simulink model "SS_IEEE_9_bus_revised_dynamicPhasor1"  (R2023b)
settings: Solver=VariableStepAuto  StartTime=0.0  StopTime=10.0  RelTol=1e-3
settings Model: Creator=dongyuli  LastModifiedBy=dongyuli

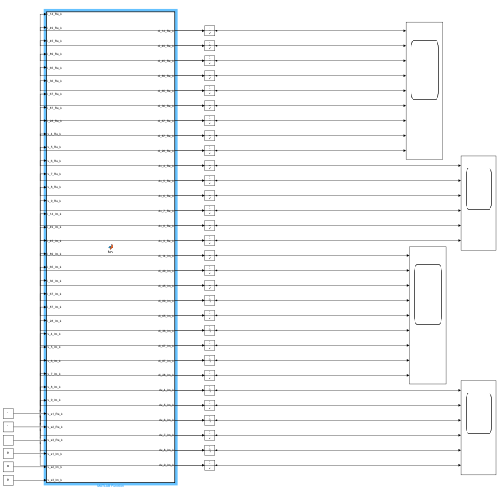
[thumbnail: Simulink's stored preview of the top-level diagram]
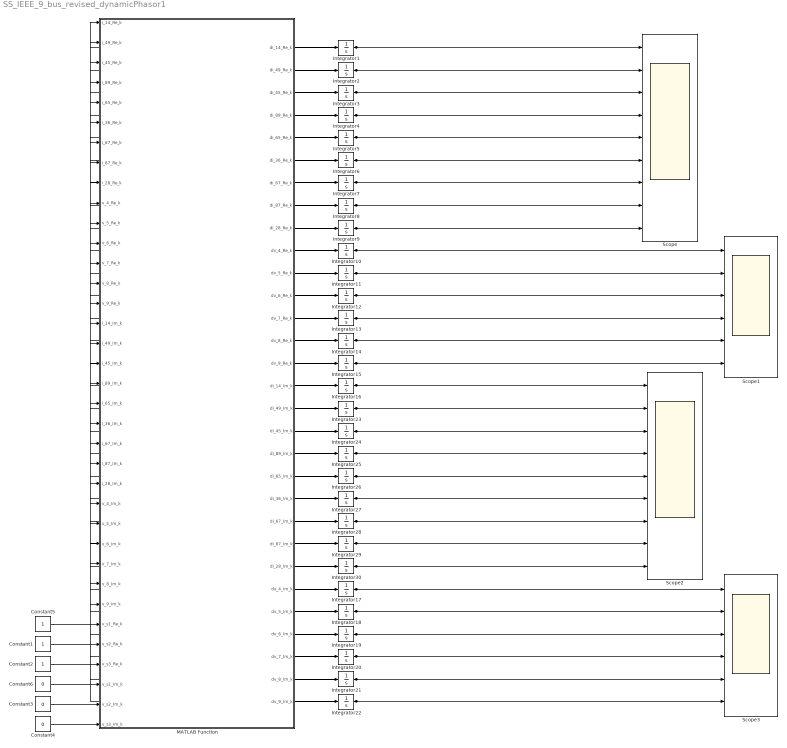
== system SS_IEEE_9_bus_revised_dynamicPhasor1 ==
  Constant1 : Constant
  Constant2 : Constant
  Constant3 : Constant  Value=0
  Constant4 : Constant  Value=0
  Constant5 : Constant
  Constant6 : Constant  Value=0
  Integrator{1..30} (30 alike) : Integrator
  MATLAB Function : MATLAB Function  TreatAsAtomicUnit=on
  Scope : Scope  NumInputPorts=9
  Scope1 : Scope  NumInputPorts=6
  Scope2 : Scope  NumInputPorts=9
  Scope3 : Scope  NumInputPorts=6
  wires:
  MATLAB Function/1(di_14_Re_k) -> Integrator1/1
  MATLAB Function/2(di_49_Re_k) -> Integrator2/1
  MATLAB Function/3(di_45_Re_k) -> Integrator3/1
  MATLAB Function/4(di_89_Re_k) -> Integrator4/1
  MATLAB Function/5(di_65_Re_k) -> Integrator5/1
  MATLAB Function/6(di_36_Re_k) -> Integrator6/1
  MATLAB Function/7(di_67_Re_k) -> Integrator7/1
  MATLAB Function/8(di_87_Re_k) -> Integrator8/1
  MATLAB Function/9(di_28_Re_k) -> Integrator9/1
  MATLAB Function/10(dv_4_Re_k) -> Integrator10/1
  MATLAB Function/11(dv_5_Re_k) -> Integrator11/1
  MATLAB Function/12(dv_6_Re_k) -> Integrator12/1
  MATLAB Function/13(dv_7_Re_k) -> Integrator13/1
  MATLAB Function/14(dv_8_Re_k) -> Integrator14/1
  MATLAB Function/15(dv_9_Re_k) -> Integrator15/1
  MATLAB Function/16(di_14_Im_k) -> Integrator16/1
  MATLAB Function/17(di_49_Im_k) -> Integrator23/1
  MATLAB Function/18(di_45_Im_k) -> Integrator24/1
  MATLAB Function/19(di_89_Im_k) -> Integrator25/1
  MATLAB Function/20(di_65_Im_k) -> Integrator26/1
  MATLAB Function/21(di_36_Im_k) -> Integrator27/1
  MATLAB Function/22(di_67_Im_k) -> Integrator28/1
  MATLAB Function/23(di_87_Im_k) -> Integrator29/1
  MATLAB Function/24(di_28_Im_k) -> Integrator30/1
  MATLAB Function/25(dv_4_Im_k) -> Integrator17/1
  MATLAB Function/26(dv_5_Im_k) -> Integrator18/1
  MATLAB Function/27(dv_6_Im_k) -> Integrator19/1
  MATLAB Function/28(dv_7_Im_k) -> Integrator20/1
  MATLAB Function/29(dv_8_Im_k) -> Integrator21/1
  MATLAB Function/30(dv_9_Im_k) -> Integrator22/1
  Integrator1/1 -> Scope/1, MATLAB Function/1(i_14_Re_k)
  Integrator2/1 -> Scope/2, MATLAB Function/2(i_49_Re_k)
  Integrator3/1 -> Scope/3, MATLAB Function/3(i_45_Re_k)
  Constant5/1 -> MATLAB Function/31(v_s1_Re_k)
  Constant1/1 -> MATLAB Function/32(v_s2_Re_k)
  Constant2/1 -> MATLAB Function/33(v_s3_Re_k)
  Integrator4/1 -> Scope/4, MATLAB Function/4(i_89_Re_k)
  Integrator5/1 -> Scope/5, MATLAB Function/5(i_65_Re_k)
  Integrator6/1 -> Scope/6, MATLAB Function/6(i_36_Re_k)
  Integrator7/1 -> Scope/7, MATLAB Function/7(i_67_Re_k)
  Integrator8/1 -> Scope/8, MATLAB Function/8(i_87_Re_k)
  Integrator9/1 -> Scope/9, MATLAB Function/9(i_28_Re_k)
  Integrator10/1 -> Scope1/1, MATLAB Function/10(v_4_Re_k)
  Integrator11/1 -> Scope1/2, MATLAB Function/11(v_5_Re_k)
  Integrator12/1 -> Scope1/3, MATLAB Function/12(v_6_Re_k)
  Integrator13/1 -> Scope1/4, MATLAB Function/13(v_7_Re_k)
  Integrator14/1 -> Scope1/5, MATLAB Function/14(v_8_Re_k)
  Integrator15/1 -> Scope1/6, MATLAB Function/15(v_9_Re_k)
  Integrator16/1 -> Scope2/1, MATLAB Function/16(i_14_Im_k)
  Integrator23/1 -> Scope2/2, MATLAB Function/17(i_49_Im_k)
  Integrator24/1 -> Scope2/3, MATLAB Function/18(i_45_Im_k)
  Integrator25/1 -> Scope2/4, MATLAB Function/19(i_89_Im_k)
  Integrator26/1 -> Scope2/5, MATLAB Function/20(i_65_Im_k)
  Integrator27/1 -> Scope2/6, MATLAB Function/21(i_36_Im_k)
  Integrator28/1 -> Scope2/7, MATLAB Function/22(i_67_Im_k)
  Integrator29/1 -> Scope2/8, MATLAB Function/23(i_87_Im_k)
  Integrator30/1 -> Scope2/9, MATLAB Function/24(i_28_Im_k)
  Integrator17/1 -> Scope3/1, MATLAB Function/25(v_4_Im_k)
  Integrator18/1 -> Scope3/2, MATLAB Function/26(v_5_Im_k)
  Integrator19/1 -> Scope3/3, MATLAB Function/27(v_6_Im_k)
  Integrator20/1 -> Scope3/4, MATLAB Function/28(v_7_Im_k)
  Integrator21/1 -> Scope3/5, MATLAB Function/29(v_8_Im_k)
  Integrator22/1 -> Scope3/6, MATLAB Function/30(v_9_Im_k)
  Constant6/1 -> MATLAB Function/34(v_s1_Im_k)
  Constant3/1 -> MATLAB Function/35(v_s2_Im_k)
  Constant4/1 -> MATLAB Function/36(v_s3_Im_k)

== matlab function SS_IEEE_9_bus_revised_dynamicPhasor1/MATLAB Function ==
  data: i_14_Re_k input; di_14_Re_k output; di_49_Re_k output; di_45_Re_k output; di_89_Re_k output; di_65_Re_k output; di_36_Re_k output; di_67_Re_k output; di_87_Re_k output; di_28_Re_k output; dv_4_Re_k output; dv_5_Re_k output; dv_6_Re_k output; dv_7_Re_k output; dv_8_Re_k output; dv_9_Re_k output; i_49_Re_k input; i_45_Re_k input; i_89_Re_k input; i_65_Re_k input; i_36_Re_k input; i_67_Re_k input; i_87_Re_k input; i_28_Re_k input; v_4_Re_k input; v_5_Re_k input; v_6_Re_k input; v_7_Re_k input; v_8_Re_k input; v_9_Re_k input; i_14_Im_k input; i_49_Im_k input; i_45_Im_k input; i_89_Im_k input; i_65_Im_k input; i_36_Im_k input; i_67_Im_k input; i_87_Im_k input; i_28_Im_k input; v_4_Im_k input; v_5_Im_k input; v_6_Im_k input; v_7_Im_k input; v_8_Im_k input; v_9_Im_k input; v_s1_Re_k input; v_s2_Re_k input; v_s3_Re_k input; di_14_Im_k output; di_49_Im_k output; di_45_Im_k output; di_89_Im_k output; di_65_Im_k output; di_36_Im_k output; di_67_Im_k output; di_87_Im_k output; di_28_Im_k output; dv_4_Im_k output; dv_5_Im_k output; dv_6_Im_k output; dv_7_Im_k output; dv_8_Im_k output; dv_9_Im_k output; v_s1_Im_k input; v_s2_Im_k input; v_s3_Im_k input
function [di_14_Re_k, di_49_Re_k, di_45_Re_k, di_89_Re_k, di_65_Re_k, di_36_Re_k, di_67_Re_k, di_87_Re_k, di_28_Re_k, dv_4_Re_k, dv_5_Re_k, dv_6_Re_k, dv_7_Re_k, dv_8_Re_k, dv_9_Re_k, di_14_Im_k, di_49_Im_k, di_45_Im_k, di_89_Im_k, di_65_Im_k, di_36_Im_k, di_67_Im_k, di_87_Im_k, di_28_Im_k, dv_4_Im_k, dv_5_Im_k, dv_6_Im_k, dv_7_Im_k, dv_8_Im_k, dv_9_Im_k] = fcn(i_14_Re_k, i_49_Re_k, i_45_Re_k, i_89_Re_k, i_65_Re_k, i_36_Re_k, i_67_Re_k, i_87_Re_k, i_28_Re_k, v_4_Re_k, v_5_Re_k, v_6_Re_k, v_7_Re_k, v_8_Re_k, v_9_Re_k, i_14_Im_k, i_49_Im_k, i_45_Im_k, i_89_Im_k, i_65_Im_k, i_36_Im_k, i_67_Im_k, i_87_Im_k, i_28_Im_k, v_4_Im_k, v_5_Im_k, v_6_Im_k, v_7_Im_k, v_8_Im_k, v_9_Im_k, v_s1_Re_k, v_s2_Re_k, v_s3_Re_k, v_s1_Im_k, v_s2_Im_k, v_s3_Im_k)

f = 50;
w = 2*pi*f;

V_base = 345;
MVA_base = 100;
Z_base = (sqrt(3)*V_base^2)/MVA_base;

R_14 = 0.01*Z_base;
R_28 = 0.01*Z_base;
R_36 = 0.01*Z_base;

R_49 = 0.01*Z_base;
R_45 = 0.017*Z_base;
R_89 = 0.032*Z_base;
R_65 = 0.039*Z_base;
R_67 = 0.0119*Z_base;
R_87 = 0.0085*Z_base;

L_14 = 0.0576*Z_base/w;
L_49 = 0.085*Z_base/w;
L_45 = 0.092*Z_base/w;
L_89 = 0.161*Z_base/w;
L_65 = 0.170*Z_base/w;
L_36 = 0.0586*Z_base/w;
L_67 = 0.1008*Z_base/w;
L_87 = 0.072*Z_base/w;
L_28 = 0.0625*Z_base/w;

L_1 = 0.0608*Z_base/w;
L_2 = 0.1198*Z_base/w;
L_3 = 0.1813*Z_base/w;

C_4 = (0.079 + 0.088)*Z_base/w;
C_5 = (0.079 + 0.179)*Z_base/w;
C_6 = (0.179 + 0.1045)*Z_base/w;
C_7 = (0.1045 + 0.0745)*Z_base/w;
C_8 = (0.0745 + 0.153)*Z_base/w;
C_9 = (0.088 + 0.153)*Z_base/w;

X = [i_14_Re_k, i_49_Re_k, i_45_Re_k, i_89_Re_k, i_65_Re_k, i_36_Re_k, i_67_Re_k, i_87_Re_k, i_28_Re_k, v_4_Re_k, v_5_Re_k, v_6_Re_k, v_7_Re_k, v_8_Re_k, v_9_Re_k, i_14_Im_k, i_49_Im_k, i_45_Im_k, i_89_Im_k, i_65_Im_k, i_36_Im_k, i_67_Im_k, i_87_Im_k, i_28_Im_k, v_4_Im_k, v_5_Im_k, v_6_Im_k, v_7_Im_k, v_8_Im_k, v_9_Im_k]';

U = [v_s1_Re_k, v_s2_Re_k, v_s3_Re_k, v_s1_Im_k, v_s2_Im_k, v_s3_Im_k]';

%A =[-R_14/L_14 0 0 0 0 0 0 0 0 1/L_14 0 0 -1/L_14 0 0 0 0 0;
%    0 -R_49/L_49 0 0 0 0 0 0 0 0 0 0 1/L_49 0 0 0 0 -1/L_49;
%    0 0 -R_45/L_45 0 0 0 0 0 0 0 0 0 1/L_45 -1/L_45 0 0 0 0;
%    0 0 0 -R_89/L_89 0 0 0 0 0 0 0 0 0 0 0 0 1/L_89 -1/L_89;
%    0 0 0 0 -R_65/L_65 0 0 0 0 0 0 0 0 -1/L_65 1/L_65 0 0 0;
%    0 0 0 0 0 -R_36/L_36 0 0 0 0 0 1/L_36 0 0 -1/L_36 0 0 0;
%    0 0 0 0 0 0 -R_67/L_67 0 0 0 0 0 0 0 1/L_67 -1/L_67 0 0;
%    0 0 0 0 0 0 0 -R_87/L_87 0 0 0 0 0 0 0 -1/L_87 1/L_87 0;
%    0 0 0 0 0 0 0 0 -R_28/L_28 0 1/L_28 0 0 0 0 0 -1/L_28 0;
%    -1/C_1 0 0 0 0 0 0 0 0 0 0 0 0 0 0 0 0 0;
%    0 0 0 0 0 0 0 0 -1/C_2 0 0 0 0 0 0 0 0 0;
%    0 0 0 0 0 -1/C_3 0 0 0 0 0 0 0 0 0 0 0 0;
%    1/C_4 -1/C_4 -1/C_4 0 0 0 0 0 0 0 0 0 0 0 0 0 0 0;
%    0 0 1/C_5 0 1/C_5 0 0 0 0 0 0 0 0 0 0 0 0 0;
%    0 0 0 0 -1/C_6 1/C_6 -1/C_6 0 0 0 0 0 0 0 0 0 0 0;
%    0 0 0 0 0 0 1/C_7 1/C_7 0 0 0 0 0 0 0 0 0 0;
%    0 0 0 -1/C_8 0 0 0 -1/C_8 1/C_8 0 0 0 0 0 0 0 0 0;
%    0 1/C_9 0 1/C_9 0 0 0 0 0 0 0 0 0 0 0 0 0 0];

A = [-R_14/(L_14+L_1) 0 0 0 0 0 0 0 0 -1/(L_14+L_1) 0 0 0 0 0;
    0 -R_49/L_49 0 0 0 0 0 0 0 1/L_49 0 0 0 0 -1/L_49;
    0 0 -R_45/L_45 0 0 0 0 0 0 1/L_45 -1/L_45 0 0 0 0;
    0 0 0 -R_89/L_89 0 0 0 0 0 0 0 0 0 1/L_89 -1/L_89;
    0 0 0 0 -R_65/L_65 0 0 0 0 0 -1/L_65 1/L_65 0 0 0;
    0 0 0 0 0 -R_36/(L_36+L_3) 0 0 0 0 0 -1/(L_36+L_3) 0 0 0;
    0 0 0 0 0 0 -R_67/L_67 0 0 0 0 1/L_67 -1/L_67 0 0;
    0 0 0 0 0 0 0 -R_87/L_87 0 0 0 0 0 -1/L_87 1/L_87;
    0 0 0 0 0 0 0 0 -R_28/(L_28+L_2) 0 0 0 0 -1/(L_28+L_2) 0;
    1/C_4 -1/C_4 -1/C_4 0 0 0 0 0 0 0 0 0 0 0 0;
    0 0 1/C_5 0 1/C_5 0 0 0 0 0 0 0 0 0 0;
    0 0 0 0 -1/C_6 1/C_6 -1/C_6 0 0 0 0 0 0 0 0;
    0 0 0 0 0 0 1/C_7 1/C_7 0 0 0 0 0 0 0;
    0 0 0 0 -1/C_8 0 0 -1/C_8 1/C_8 0 0 0 0 0 0;
    0 1/C_9 0 1/C_9 0 0 0 0 0 0 0 0 0 0 0];

I = eye(15);

k = 1;

A_k = [A k*w*I;
      -k*w*I A];

B =[1/(L_14+L_1) 0 0;
    0 0 0;
    0 0 0;
    0 0 0;
    0 0 0;
    0 0 1/(L_36+L_3);
    0 0 0;
    0 0 0;
    0 1/(L_28+L_2) 0;
    0 0 0;
    0 0 0;
    0 0 0;
    0 0 0;
    0 0 0;
    0 0 0];

O = zeros(15,3);

B_k = [B O;
       O B];

dX = A_k*X + B_k*U;

di_14_Re_k = dX(1);
di_49_Re_k = dX(2);
di_45_Re_k = dX(3);
di_89_Re_k = dX(4);
di_65_Re_k = dX(5);
di_36_Re_k = dX(6);
di_67_Re_k = dX(7);
di_87_Re_k = dX(8);
di_28_Re_k = dX(9);

dv_4_Re_k = dX(10);
dv_5_Re_k = dX(11);
dv_6_Re_k = dX(12);
dv_7_Re_k = dX(13);
dv_8_Re_k = dX(14);
dv_9_Re_k = dX(15);

di_14_Im_k = dX(16);
di_49_Im_k = dX(17);
di_45_Im_k = dX(18);
di_89_Im_k = dX(19);
di_65_Im_k = dX(20);
di_36_Im_k = dX(21);
di_67_Im_k = dX(22);
di_87_Im_k = dX(23);
di_28_Im_k = dX(24);

dv_4_Im_k = dX(25);
dv_5_Im_k = dX(26);
dv_6_Im_k = dX(27);
dv_7_Im_k = dX(28);
dv_8_Im_k = dX(29);
dv_9_Im_k = dX(30);

end
